simulink model "planetary_phase"  (R2023b)
settings: Solver=ode4  StartTime=0.0  StopTime=T  FixedStep=step_t  RelTol=1e-3
values from neighbouring files (symbols this model uses):
  a0 = (mu*T^2/(4*pi^2))^(1/3)    [planetary_phase_script.m]    (also in script_jupiter.m)
  A0 = [1 0 0; 0 0 1; 0 -1 0]*[0 0 1; 0 1 0; -1 0 0]    [planetary_phase_script.m]    (also in script_aocs.m = [0 0 1; 0 1 0; -1 0 0]; script_jupiter.m; simulation_inner1.m = A_b_n(:,:,end); srp_interplanetary.m = A_b_n(:,:,end))
  braccio_x = 2.7    [planetary_phase_script.m]    (also in script_aocs.m; script_jupiter.m; simulation_inner1.m; srp_interplanetary.m)
  braccio_y = 2.7    [planetary_phase_script.m]    (also in script_aocs.m; script_jupiter.m; simulation_inner1.m; srp_interplanetary.m)
  braccio_z = 3.2    [planetary_phase_script.m]    (also in script_aocs.m; script_jupiter.m; simulation_inner1.m; srp_interplanetary.m)
  dist = 1    [planetary_phase_script.m]    (also in script_jupiter.m)
  e0 = 1 - rp/a0    [planetary_phase_script.m]    (also in script_jupiter.m)
  gain_alphas = [-1000; -1000; -10]    [planetary_phase_script.m]    (also in script_aocs.m = [-100 -100 -1]'; script_jupiter.m; simulation_inner1.m = [-100 -100 -1]'; srp_interplanetary.m = [-100 -100 -1]')
  gain_omega = -1    [planetary_phase_script.m]    (also in script_aocs.m = -950; script_jupiter.m; simulation_inner1.m = -950; srp_interplanetary.m = -950)
  I = diag([11245.08 10044.71 17593.63])    [planetary_phase_script.m]    (also in script_aocs.m = [11245.08 0 0; 0 10044.71 0; 0 0 17593.63]; script_jupiter.m; simulation_inner1.m = [11245.08 0 0; 0 10044.71 0; 0 0 17593.63]; srp_interplanetary.m = [11245.08 0 0; 0 10044.71 0; 0 0 17593.63])
  i0 = el(3)    [planetary_phase_script.m]    (also in script_jupiter.m)
  I_inv = inv(I)    [planetary_phase_script.m]    (also in script_aocs.m; script_jupiter.m; simulation_inner1.m; srp_interplanetary.m)
  j_b = [0.05; 0.05; 0.05]    [planetary_phase_script.m]    (also in script_jupiter.m)
  mu = astroConstants(4)    [calcolo_distanze.m]    (also in loadData.m; loadData_ore.m; planetary_phase_script.m = astroConstants(15); script_aocs.m)
  n = 2 * 2 * pi/60    (= 0.209439510239)    [planetary_phase_script.m]    (also in script_aocs.m = 0.10471975512; script_jupiter.m; simulation_inner1.m = 0.10471975512; srp_interplanetary.m = 0.10471975512)
  th0 = deg2rad(180)    [planetary_phase_script.m]    (also in script_jupiter.m)
  toll = deg2rad(15)    [planetary_phase_script.m]    (also in script_aocs.m; script_jupiter.m; simulation_inner1.m; srp_interplanetary.m)
  w0 = [0 0 n]    [planetary_phase_script.m]    (also in script_aocs.m; script_jupiter.m; simulation_inner1.m = w(:,end); srp_interplanetary.m = w(:,end))
undefined symbols (not defined in the file or in its folder): D, N
libraries: matrix_library x3, simulink x3, vrlib x1
(part 2 of 2)

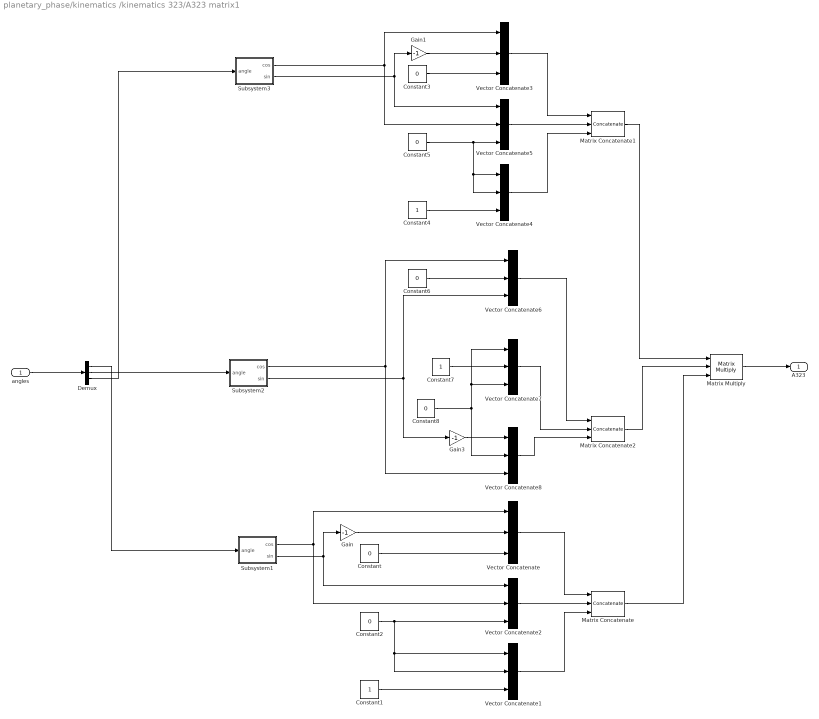
== system planetary_phase/kinematics /kinematics 323/A323 matrix1 ==
  angles : Inport
  Constant{,2..3,5..6,8} (6 alike) : Constant  Value=0
  Constant1 : Constant
  Constant4 : Constant
  Constant7 : Constant
  Demux : Demux  Outputs=3
  Gain : Gain  Gain=-1
  Gain1 : Gain  Gain=-1
  Gain3 : Gain  Gain=-1
  Matrix Concatenate : Concatenate  NumInputs=3  Mode=Multidimensional array  ConcatenateDimension=2
  Matrix Concatenate1 : Concatenate  NumInputs=3  Mode=Multidimensional array  ConcatenateDimension=2
  Matrix Concatenate2 : Concatenate  NumInputs=3  Mode=Multidimensional array  ConcatenateDimension=2
  Matrix Multiply : Product  Inputs=3  Multiplication=Matrix(*)
  Subsystem1 : Subsystem
  Subsystem2 : Subsystem
  Subsystem3 : Subsystem
  Vector Concatenate{,1..8} (9 alike) : Concatenate  NumInputs=3
  A323 : Outport
  wires:
  angles/1 -> Demux/1
  Demux/1 -> Subsystem1/1(angle)
  Demux/2 -> Subsystem2/1(angle)
  Demux/3 -> Subsystem3/1(angle)
  Gain3/1 -> Vector Concatenate8/1
  Constant8/1 -> Vector Concatenate8/2, Vector Concatenate7/3, Vector Concatenate7/1
  Constant7/1 -> Vector Concatenate7/2
  Subsystem2/2(sin) -> Gain3/1, Vector Concatenate6/3
  Constant6/1 -> Vector Concatenate6/2
  Subsystem2/1(cos) -> Vector Concatenate6/1, Vector Concatenate8/3
  Vector Concatenate8/1 -> Matrix Concatenate2/3
  Vector Concatenate7/1 -> Matrix Concatenate2/2
  Vector Concatenate6/1 -> Matrix Concatenate2/1
  Matrix Multiply/1 -> A323/1
  Matrix Concatenate1/1 -> Matrix Multiply/1
  Matrix Concatenate/1 -> Matrix Multiply/3
  Matrix Concatenate2/1 -> Matrix Multiply/2
  Subsystem3/2(sin) -> Gain1/1, Vector Concatenate5/1
  Subsystem3/1(cos) -> Vector Concatenate5/2, Vector Concatenate3/1
  Constant4/1 -> Vector Concatenate4/3
  Gain1/1 -> Vector Concatenate3/2
  Constant3/1 -> Vector Concatenate3/3
  Constant5/1 -> Vector Concatenate4/2, Vector Concatenate4/1, Vector Concatenate5/3
  Vector Concatenate3/1 -> Matrix Concatenate1/1
  Vector Concatenate5/1 -> Matrix Concatenate1/2
  Vector Concatenate4/1 -> Matrix Concatenate1/3
  Vector Concatenate1/1 -> Matrix Concatenate/3
  Vector Concatenate2/1 -> Matrix Concatenate/2
  Vector Concatenate/1 -> Matrix Concatenate/1
  Constant2/1 -> Vector Concatenate2/3, Vector Concatenate1/2, Vector Concatenate1/1
  Constant/1 -> Vector Concatenate/3
  Gain/1 -> Vector Concatenate/2
  Constant1/1 -> Vector Concatenate1/3
  Subsystem1/1(cos) -> Vector Concatenate/1, Vector Concatenate2/2
  Subsystem1/2(sin) -> Vector Concatenate2/1, Gain/1

== system planetary_phase/kinematics /logic 323/Subsystem4 ==
  In2 : Inport
  In1 : Inport  Port=2
  In4 : Inport  Port=3
  In3 : Inport  Port=4
  Constant : Constant
  Constant1 : Constant
  Constant2 : Constant  Value=0
  Constant3 : Constant  Value=0
  Data Type Conversion : DataTypeConversion  OutDataTypeStr=boolean  SaturateOnIntegerOverflow=off  RndMeth=Floor
  If Action Subsystem : Subsystem  TreatAsAtomicUnit=on
  If Action Subsystem1 : Subsystem  TreatAsAtomicUnit=on
  If Action Subsystem2 : Subsystem  TreatAsAtomicUnit=on
  If Action Subsystem3 : Subsystem  TreatAsAtomicUnit=on
  If2 : If  NumInputs=4  IfExpression=u1 == 1  ElseIfExpressions=u1 == 0 & u3 == 0 & u4 == 1, u1 == 0 & u2 == 0 & u3 == 1 & u4 == 0
  Merge : Merge  Inputs=4
  Out1 : Outport
  wires:
  If2/1 -> If Action Subsystem/Action
  If2/2 -> If Action Subsystem1/Action
  If2/3 -> If Action Subsystem2/Action
  If2/4 -> If Action Subsystem3/Action
  Constant/1 -> If Action Subsystem/1(In1)
  Constant1/1 -> If Action Subsystem1/1(In1)
  Constant2/1 -> If Action Subsystem2/1(In1)
  Constant3/1 -> If Action Subsystem3/1(In1)
  If Action Subsystem/1(Out1) -> Merge/1
  If Action Subsystem1/1(Out1) -> Merge/2
  If Action Subsystem2/1(Out1) -> Merge/3
  If Action Subsystem3/1(Out1) -> Merge/4
  Merge/1 -> Data Type Conversion/1
  Data Type Conversion/1 -> Out1/1
  In1/1 -> If2/1
  In2/1 -> If2/2
  In3/1 -> If2/3
  In4/1 -> If2/4

== system planetary_phase/Disturbances/Disturbances/Gravity gradient Torque/Inertial to LVLH Matrix ==
  th : Inport
  i : Inport  Port=2
  Constant1 : Constant  Value=[0 0 -1; 0 1 0;1 0 0]'
  MatrixMultiply : Product  Multiplication=Matrix(*)
  Rotation matrix i : Subsystem
  Rotation matrix n : Subsystem
  A_L/N : Outport
  wires:
  th/1 -> Rotation matrix n/1(th)
  i/1 -> Rotation matrix i/1(i)
  MatrixMultiply/1 -> A_L/N/1
  Rotation matrix n/1(R_n) -> MatrixMultiply/1
  Rotation matrix i/1(R_i) -> MatrixMultiply/2

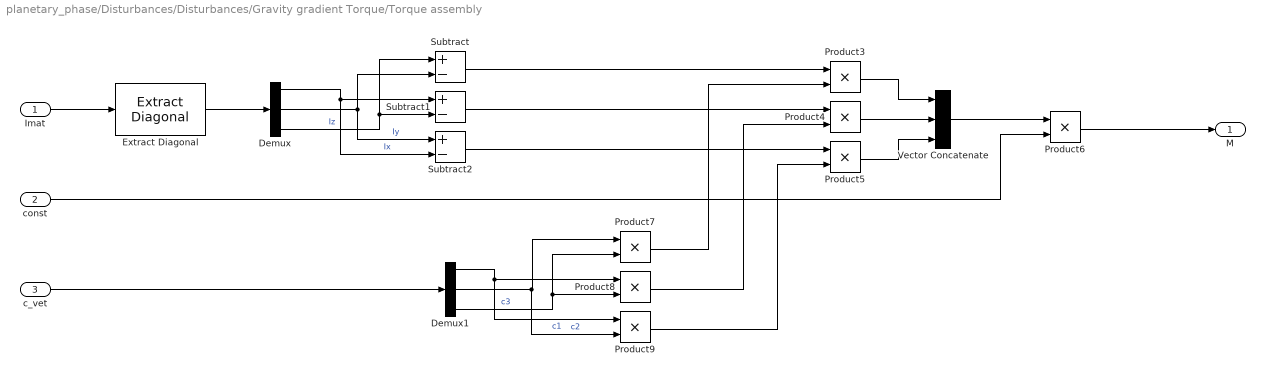
== system planetary_phase/Disturbances/Disturbances/Gravity gradient Torque/Torque assembly ==
  Imat : Inport
  const : Inport  Port=2
  c_vet : Inport  Port=3
  Demux : Demux  Outputs=3
  Demux1 : Demux  Outputs=3
  Extract Diagonal : matrix_library/Extract Diagonal
      settings: LibrarySourceBlock=|
      | simulink/Matrix
      | Operations/Extract Diagonal
  Product{3..9} (7 alike) : Product
  Subtract : Sum  Inputs=+-
  Subtract1 : Sum  Inputs=+-
  Subtract2 : Sum  Inputs=+-
  Vector Concatenate : Concatenate  NumInputs=3
  M : Outport
  wires:
  Imat/1 -> Extract Diagonal/1
  Extract Diagonal/1 -> Demux/1
  Demux/1 -> Subtract1/1, Subtract2/2  "Ix"
  c_vet/1 -> Demux1/1
  const/1 -> Product6/2
  Demux/2 -> Subtract/2, Subtract2/1  "Iy"
  Demux/3 -> Subtract/1, Subtract1/2  "Iz"
  Product4/1 -> Vector Concatenate/2
  Product3/1 -> Vector Concatenate/1
  Product5/1 -> Vector Concatenate/3
  Vector Concatenate/1 -> Product6/1
  Product6/1 -> M/1
  Demux1/1 -> Product9/1, Product8/1  "c1"
  Demux1/2 -> Product9/2, Product7/1  "c2"
  Demux1/3 -> Product8/2, Product7/2  "c3"
  Product7/1 -> Product3/2
  Product8/1 -> Product4/2
  Product9/1 -> Product5/2
  Subtract/1 -> Product3/1
  Subtract1/1 -> Product4/1
  Subtract2/1 -> Product5/1

== system planetary_phase/Disturbances/Disturbances/Magnetic field torque/Norm ==
  1 : Inport
  Dot Product : DotProduct  OutDataTypeStr=Inherit: Inherit via internal rule
  Sqrt : Sqrt
  Output : Outport
  wires:
  1/1 -> Dot Product/1, Dot Product/2
  Dot Product/1 -> Sqrt/1
  Sqrt/1 -> Output/1

== system planetary_phase/Disturbances/Disturbances/SRP Torque/Illumination check ==
  1 : Inport
  Constant : Constant  Value=0
  Less Than : RelationalOperator  Operator=>  OutDataTypeStr=boolean  RndMeth=Simplest  InputSameDT=off
  Product6 : Product
  Out1 : Outport
  wires:
  1/1 -> Less Than/1, Product6/1
  Less Than/1 -> Product6/2
  Constant/1 -> Less Than/2
  Product6/1 -> Out1/1

== system planetary_phase/Disturbances/Disturbances/SRP Torque/Normalize ==
  In1 : Inport
  Divide : Product  Inputs=*/
  Divide1 : Product  Inputs=*/
  Divide2 : Product  Inputs=*/
  Selector : Selector  NumberOfDimensions=2  InputPortWidth=3  IndexOptions=Select all,Index vector (dialog)  Indices=[1 3],1  OutputSizes=1,1
  Selector2 : Selector  NumberOfDimensions=2  InputPortWidth=3  IndexOptions=Select all,Index vector (dialog)  Indices=1:N,2  OutputSizes=1,1
  Selector6 : Selector  NumberOfDimensions=2  InputPortWidth=3  IndexOptions=Select all,Index vector (dialog)  Indices=1:N,3  OutputSizes=1,1
  Sqrt : Sqrt
  Square : Math  Operator=square
  Square1 : Math  Operator=square
  Square2 : Math  Operator=square
  Subtract : Sum  Inputs=+++
  Output : Outport
  Output1 : Outport  Port=2
  Output2 : Outport  Port=3
  wires:
  In1/1 -> Selector/1, Selector6/1, Selector2/1  "N_b"
  Selector/1 -> Square/1, Divide/1  "N_b_x"
  Selector2/1 -> Square1/1, Divide1/1  "N_b_y"
  Selector6/1 -> Divide2/1, Square2/1  "N_b_z"
  Square1/1 -> Subtract/2
  Square/1 -> Subtract/1
  Square2/1 -> Subtract/3
  Subtract/1 -> Sqrt/1
  Sqrt/1 -> Divide2/2, Divide/2, Divide1/2
  Divide/1 -> Output/1
  Divide1/1 -> Output1/1
  Divide2/1 -> Output2/1

== system planetary_phase/kinematics /312 Logic/Subsystem3/If Action Subsystem ==
  In1 : Inport
  Action Port : ActionPort  ActionPortLabel=if(u1 == 1)
  Out1 : Outport
  wires:
  In1/1 -> Out1/1

== system planetary_phase/kinematics /312 Logic/Subsystem3/If Action Subsystem1 ==
  In1 : Inport
  Action Port : ActionPort  ActionPortLabel=elseif(u1 == 0 & u2 == 1 & u3 == 1)
  Out1 : Outport
  wires:
  In1/1 -> Out1/1

== system planetary_phase/kinematics /312 Logic/Subsystem3/If Action Subsystem2 ==
  In1 : Inport
  Action Port : ActionPort  ActionPortLabel=elseif( u1 == 0 & u2 == 1 & u3 == 0)
  Out1 : Outport
  wires:
  In1/1 -> Out1/1

== system planetary_phase/kinematics /312 Logic/Subsystem3/If Action Subsystem3 ==
  In1 : Inport
  Action Port : ActionPort  ActionPortLabel=else
  Out1 : Outport
  wires:
  In1/1 -> Out1/1

== system planetary_phase/kinematics /angles 312 new/A323 matrix/Subsystem1 ==
  angle : Inport
  Cos : Trigonometry  Operator=cos
  Sin : Trigonometry
  cos : Outport
  sin : Outport  Port=2
  wires:
  angle/1 -> Cos/1, Sin/1
  Sin/1 -> sin/1
  Cos/1 -> cos/1

== system planetary_phase/kinematics /angles 312 new/A323 matrix/Subsystem2 ==
  angle : Inport
  Cos : Trigonometry  Operator=cos
  Sin : Trigonometry
  cos : Outport
  sin : Outport  Port=2
  wires:
  angle/1 -> Cos/1, Sin/1
  Sin/1 -> sin/1
  Cos/1 -> cos/1

== system planetary_phase/kinematics /angles 312 new/A323 matrix/Subsystem3 ==
  angle : Inport
  Cos : Trigonometry  Operator=cos
  Sin : Trigonometry
  cos : Outport
  sin : Outport  Port=2
  wires:
  Cos/1 -> cos/1
  Sin/1 -> sin/1
  angle/1 -> Sin/1, Cos/1

== system planetary_phase/kinematics /angles 323 new/Rotation 312 matrix2/Subsystem ==
  angle : Inport
  Cos : Trigonometry  Operator=cos
  Sin : Trigonometry
  cos : Outport
  sin : Outport  Port=2
  wires:
  Cos/1 -> cos/1
  Sin/1 -> sin/1
  angle/1 -> Sin/1, Cos/1

== system planetary_phase/kinematics /angles 323 new/Rotation 312 matrix2/Subsystem1 ==
  angle : Inport
  Cos : Trigonometry  Operator=cos
  Sin : Trigonometry
  cos : Outport
  sin : Outport  Port=2
  wires:
  angle/1 -> Cos/1, Sin/1
  Sin/1 -> sin/1
  Cos/1 -> cos/1

== system planetary_phase/kinematics /angles 323 new/Rotation 312 matrix2/Subsystem2 ==
  angle : Inport
  Cos : Trigonometry  Operator=cos
  Sin : Trigonometry
  cos : Outport
  sin : Outport  Port=2
  wires:
  Cos/1 -> cos/1
  Sin/1 -> sin/1
  angle/1 -> Sin/1, Cos/1

== system planetary_phase/kinematics /angles 323 new/Rotation 312 matrix2/column 1 ==
  phi : Inport
  phi2 : Inport  Port=2
  theta : Inport  Port=3
  theta2 : Inport  Port=4
  psi : Inport  Port=5
  psi2 : Inport  Port=6
  Add : Sum  Inputs=+-
  Add1 : Sum
  Gain : Gain  Gain=-1
  Product : Product
  Product1 : Product  Inputs=3
  Product2 : Product
  Product3 : Product
  Product4 : Product  Inputs=3
  Vector Concatenate : Concatenate  NumInputs=3
  Out1 : Outport
  wires:
  Add1/1 -> Vector Concatenate/3
  psi/1 -> Product/1, Product4/3
  theta2/1 -> Product4/2, Product1/2
  phi2/1 -> Product4/1, Gain/1, Product1/3
  psi2/1 -> Product3/1, Product1/1
  Gain/1 -> Product2/1
  phi/1 -> Product3/2, Product/2
  Product3/1 -> Add1/1
  Product1/1 -> Add/2
  Product2/1 -> Vector Concatenate/2
  Vector Concatenate/1 -> Out1/1
  Product/1 -> Add/1
  Add/1 -> Vector Concatenate/1
  Product4/1 -> Add1/2
  theta/1 -> Product2/2

== system planetary_phase/kinematics /angles 323 new/Rotation 312 matrix2/column 2 ==
  phi : Inport
  phi2 : Inport  Port=2
  theta : Inport  Port=3
  theta2 : Inport  Port=4
  psi : Inport  Port=5
  psi2 : Inport  Port=6
  Add : Sum
  Add1 : Sum  Inputs=+-
  Product : Product
  Product1 : Product  Inputs=3
  Product2 : Product
  Product3 : Product
  Product4 : Product  Inputs=3
  Vector Concatenate : Concatenate  NumInputs=3
  Out1 : Outport
  wires:
  Add1/1 -> Vector Concatenate/3
  theta2/1 -> Product4/3, Product1/1
  phi/1 -> Product4/2, Product2/1, Product1/3
  Product3/1 -> Add1/1
  Add/1 -> Vector Concatenate/1
  Product4/1 -> Add1/2
  Product2/1 -> Vector Concatenate/2
  Product1/1 -> Add/2
  phi2/1 -> Product3/2, Product/1
  Product/1 -> Add/1
  Vector Concatenate/1 -> Out1/1
  theta/1 -> Product2/2
  psi/1 -> Product4/1, Product/2
  psi2/1 -> Product3/1, Product1/2

== system planetary_phase/kinematics /angles 323 new/Rotation 312 matrix2/column 3 ==
  theta : Inport
  theta2 : Inport  Port=2
  psi : Inport  Port=3
  psi2 : Inport  Port=4
  Gain : Gain  Gain=-1
  Product : Product
  Product1 : Product
  Vector Concatenate : Concatenate  NumInputs=3
  Out1 : Outport
  wires:
  Product/1 -> Gain/1
  theta/1 -> Product1/1, Product/2
  Gain/1 -> Vector Concatenate/1
  psi2/1 -> Product/1
  Product1/1 -> Vector Concatenate/3
  theta2/1 -> Vector Concatenate/2
  psi/1 -> Product1/2
  Vector Concatenate/1 -> Out1/1

== system planetary_phase/kinematics /kinematics 312/Rotation 312 matrix1/Subsystem ==
  angle : Inport
  Cos : Trigonometry  Operator=cos
  Sin : Trigonometry
  cos : Outport
  sin : Outport  Port=2
  wires:
  angle/1 -> Cos/1, Sin/1
  Sin/1 -> sin/1
  Cos/1 -> cos/1

== system planetary_phase/kinematics /kinematics 312/Rotation 312 matrix1/Subsystem1 ==
  angle : Inport
  Cos : Trigonometry  Operator=cos
  Sin : Trigonometry
  cos : Outport
  sin : Outport  Port=2
  wires:
  Cos/1 -> cos/1
  Sin/1 -> sin/1
  angle/1 -> Sin/1, Cos/1

== system planetary_phase/kinematics /kinematics 312/Rotation 312 matrix1/Subsystem2 ==
  angle : Inport
  Cos : Trigonometry  Operator=cos
  Sin : Trigonometry
  cos : Outport
  sin : Outport  Port=2
  wires:
  angle/1 -> Cos/1, Sin/1
  Sin/1 -> sin/1
  Cos/1 -> cos/1

== system planetary_phase/kinematics /kinematics 312/Rotation 312 matrix1/column 1 ==
  phi : Inport
  phi2 : Inport  Port=2
  theta : Inport  Port=3
  theta2 : Inport  Port=4
  psi : Inport  Port=5
  psi2 : Inport  Port=6
  Add : Sum  Inputs=+-
  Add1 : Sum
  Gain : Gain  Gain=-1
  Product : Product
  Product1 : Product  Inputs=3
  Product2 : Product
  Product3 : Product
  Product4 : Product  Inputs=3
  Vector Concatenate : Concatenate  NumInputs=3
  Out1 : Outport
  wires:
  theta/1 -> Product2/2
  Product4/1 -> Add1/2
  Add/1 -> Vector Concatenate/1
  Product/1 -> Add/1
  Vector Concatenate/1 -> Out1/1
  Product2/1 -> Vector Concatenate/2
  Product1/1 -> Add/2
  Product3/1 -> Add1/1
  phi/1 -> Product/2, Product3/2
  Gain/1 -> Product2/1
  psi2/1 -> Product1/1, Product3/1
  phi2/1 -> Product1/3, Gain/1, Product4/1
  theta2/1 -> Product1/2, Product4/2
  psi/1 -> Product4/3, Product/1
  Add1/1 -> Vector Concatenate/3

== system planetary_phase/kinematics /kinematics 312/Rotation 312 matrix1/column 2 ==
  phi : Inport
  phi2 : Inport  Port=2
  theta : Inport  Port=3
  theta2 : Inport  Port=4
  psi : Inport  Port=5
  psi2 : Inport  Port=6
  Add : Sum
  Add1 : Sum  Inputs=+-
  Product : Product
  Product1 : Product  Inputs=3
  Product2 : Product
  Product3 : Product
  Product4 : Product  Inputs=3
  Vector Concatenate : Concatenate  NumInputs=3
  Out1 : Outport
  wires:
  psi2/1 -> Product1/2, Product3/1
  psi/1 -> Product/2, Product4/1
  theta/1 -> Product2/2
  Vector Concatenate/1 -> Out1/1
  Product/1 -> Add/1
  phi2/1 -> Product/1, Product3/2
  Product1/1 -> Add/2
  Product2/1 -> Vector Concatenate/2
  Product4/1 -> Add1/2
  Add/1 -> Vector Concatenate/1
  Product3/1 -> Add1/1
  phi/1 -> Product1/3, Product2/1, Product4/2
  theta2/1 -> Product1/1, Product4/3
  Add1/1 -> Vector Concatenate/3

== system planetary_phase/kinematics /kinematics 312/Rotation 312 matrix1/column 3 ==
  theta : Inport
  theta2 : Inport  Port=2
  psi : Inport  Port=3
  psi2 : Inport  Port=4
  Gain : Gain  Gain=-1
  Product : Product
  Product1 : Product
  Vector Concatenate : Concatenate  NumInputs=3
  Out1 : Outport
  wires:
  Vector Concatenate/1 -> Out1/1
  psi/1 -> Product1/2
  theta2/1 -> Vector Concatenate/2
  Product1/1 -> Vector Concatenate/3
  psi2/1 -> Product/1
  Gain/1 -> Vector Concatenate/1
  theta/1 -> Product/2, Product1/1
  Product/1 -> Gain/1

== system planetary_phase/kinematics /kinematics 323/A323 matrix1/Subsystem1 ==
  angle : Inport
  Cos : Trigonometry  Operator=cos
  Sin : Trigonometry
  cos : Outport
  sin : Outport  Port=2
  wires:
  Cos/1 -> cos/1
  Sin/1 -> sin/1
  angle/1 -> Sin/1, Cos/1

== system planetary_phase/kinematics /kinematics 323/A323 matrix1/Subsystem2 ==
  angle : Inport
  Cos : Trigonometry  Operator=cos
  Sin : Trigonometry
  cos : Outport
  sin : Outport  Port=2
  wires:
  Cos/1 -> cos/1
  Sin/1 -> sin/1
  angle/1 -> Sin/1, Cos/1

== system planetary_phase/kinematics /kinematics 323/A323 matrix1/Subsystem3 ==
  angle : Inport
  Cos : Trigonometry  Operator=cos
  Sin : Trigonometry
  cos : Outport
  sin : Outport  Port=2
  wires:
  angle/1 -> Cos/1, Sin/1
  Sin/1 -> sin/1
  Cos/1 -> cos/1

== system planetary_phase/kinematics /logic 323/Subsystem4/If Action Subsystem ==
  In1 : Inport
  Action Port : ActionPort  ActionPortLabel=if(u1 == 1)
  Out1 : Outport
  wires:
  In1/1 -> Out1/1

== system planetary_phase/kinematics /logic 323/Subsystem4/If Action Subsystem1 ==
  In1 : Inport
  Action Port : ActionPort  ActionPortLabel=elseif(u1 == 0 & u3 == 0 & u4 == 1)
  Out1 : Outport
  wires:
  In1/1 -> Out1/1

== system planetary_phase/kinematics /logic 323/Subsystem4/If Action Subsystem2 ==
  In1 : Inport
  Action Port : ActionPort  ActionPortLabel=elseif( u1 == 0 & u2 == 0 & u3 == 1 & u4 == 0)
  Out1 : Outport
  wires:
  In1/1 -> Out1/1

== system planetary_phase/kinematics /logic 323/Subsystem4/If Action Subsystem3 ==
  In1 : Inport
  Action Port : ActionPort  ActionPortLabel=else
  Out1 : Outport
  wires:
  In1/1 -> Out1/1

== system planetary_phase/Disturbances/Disturbances/Gravity gradient Torque/Inertial to LVLH Matrix/Rotation matrix i ==
  i : Inport
  Constant : Constant
  Constant1 : Constant  Value=0
  Cos : Trigonometry  Operator=cos
  Gain1 : Gain  Gain=-1
  Sin : Trigonometry
  Vector Concatenate4 : Concatenate  NumInputs=3
  Vector Concatenate5 : Concatenate  NumInputs=3
  Vector Concatenate6 : Concatenate  NumInputs=3
  Vector Concatenate7 : Concatenate  NumInputs=3  Mode=Multidimensional array  ConcatenateDimension=2
  R_i : Outport
  wires:
  i/1 -> Cos/1, Sin/1
  Gain1/1 -> Vector Concatenate6/2
  Constant1/1 -> Vector Concatenate4/3, Vector Concatenate4/2, Vector Concatenate5/1, Vector Concatenate6/1
  Sin/1 -> Gain1/1, Vector Concatenate5/3
  Cos/1 -> Vector Concatenate6/3, Vector Concatenate5/2
  Vector Concatenate7/1 -> R_i/1
  Constant/1 -> Vector Concatenate4/1
  Vector Concatenate4/1 -> Vector Concatenate7/1
  Vector Concatenate5/1 -> Vector Concatenate7/2
  Vector Concatenate6/1 -> Vector Concatenate7/3

== system planetary_phase/Disturbances/Disturbances/Gravity gradient Torque/Inertial to LVLH Matrix/Rotation matrix n ==
  th : Inport
  Constant : Constant  Value=0
  Constant1 : Constant
  Cos : Trigonometry  Operator=cos
  Gain1 : Gain  Gain=-1
  Sin : Trigonometry
  Vector Concatenate4 : Concatenate  NumInputs=3
  Vector Concatenate5 : Concatenate  NumInputs=3
  Vector Concatenate6 : Concatenate  NumInputs=3
  Vector Concatenate7 : Concatenate  NumInputs=3  Mode=Multidimensional array  ConcatenateDimension=2
  R_n : Outport
  wires:
  Constant/1 -> Vector Concatenate6/1, Vector Concatenate6/2, Vector Concatenate5/3, Vector Concatenate4/3
  Sin/1 -> Vector Concatenate4/2, Gain1/1
  Cos/1 -> Vector Concatenate4/1, Vector Concatenate5/2
  Constant1/1 -> Vector Concatenate6/3
  Vector Concatenate6/1 -> Vector Concatenate7/3
  Vector Concatenate4/1 -> Vector Concatenate7/1
  Vector Concatenate5/1 -> Vector Concatenate7/2
  Vector Concatenate7/1 -> R_n/1
  Gain1/1 -> Vector Concatenate5/1
  th/1 -> Cos/1, Sin/1
